simulink model "Neurofeedback_Draft_Models"  (R2022a)
settings: Solver=VariableStepAuto  StartTime=0.0  StopTime=10.0  RelTol=1e-3
settings Model: Creator=mariodelossantos  LastModifiedBy=mdls3

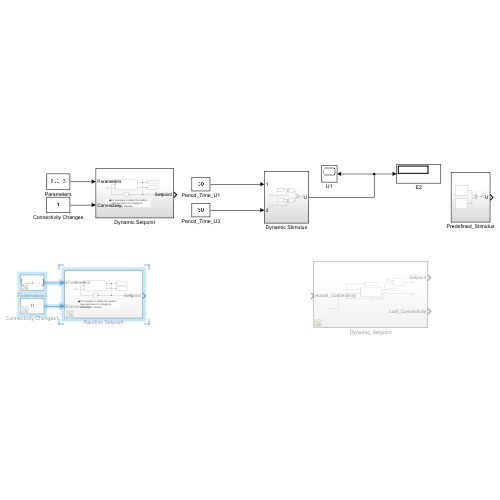
[thumbnail: Simulink's stored preview of the top-level diagram]
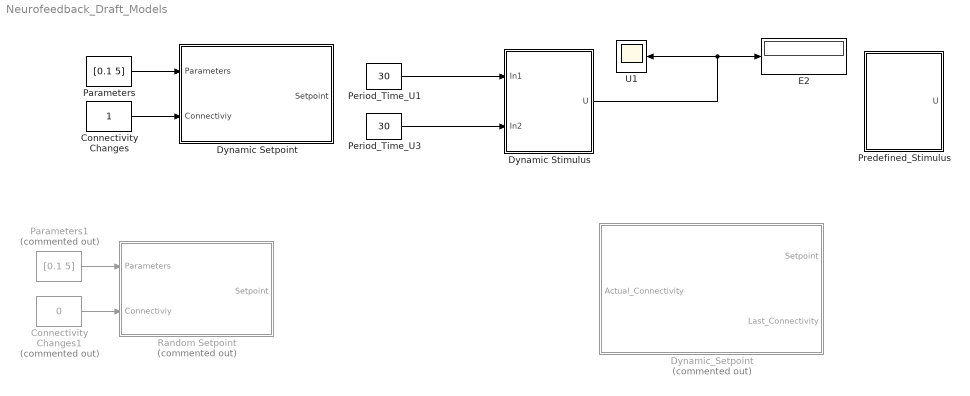
== system Neurofeedback_Draft_Models ==
  Connectivity Changes : Constant
  Connectivity Changes1 : Constant  Commented=on  Value=0
  Dynamic Setpoint : Subsystem
  Dynamic Stimulus : Subsystem
  Dynamic_Setpoint : Subsystem  Commented=on
  E2 : Display
  Parameters : Constant  Value=[0.1 5]
  Parameters1 : Constant  Commented=on  Value=[0.1 5]
  Period_Time_U1 : Constant  Value=30
  Period_Time_U3 : Constant  Value=30
  Predefined_Stimulus : Subsystem
  Random Setpoint : Subsystem  Commented=on
  U1 : Scope
  wires:
  Parameters/1 -> Dynamic Setpoint/1(Parameters)
  Connectivity Changes/1 -> Dynamic Setpoint/2(Connectiviy)
  Period_Time_U1/1 -> Dynamic Stimulus/1(In1)
  Period_Time_U3/1 -> Dynamic Stimulus/2(In2)
  Dynamic Stimulus/1(U) -> E2/1, U1/1
  Connectivity Changes1/1 -> Random Setpoint/2(Connectiviy)
  Parameters1/1 -> Random Setpoint/1(Parameters)

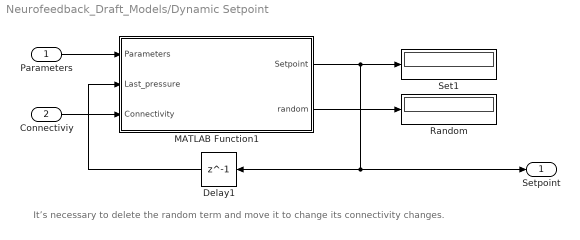
== system Neurofeedback_Draft_Models/Dynamic Setpoint ==
  note: It’s necessary to delete the random term and move it to change its connectivity changes.
  Parameters : Inport
  Connectiviy : Inport  Port=2
  Delay1 : Delay  DelayLength=1  InitialCondition=0
  MATLAB Function1 : MATLAB Function  TreatAsAtomicUnit=on
  Random : Display
  Set1 : Display
  Setpoint : Outport
  wires:
  Parameters/1 -> MATLAB Function1/1(Parameters)
  MATLAB Function1/2(random) -> Random/1
  MATLAB Function1/1(Setpoint) -> Set1/1, Setpoint/1, Delay1/1
  Delay1/1 -> MATLAB Function1/2(Last_pressure)
  Connectiviy/1 -> MATLAB Function1/3(Connectivity)

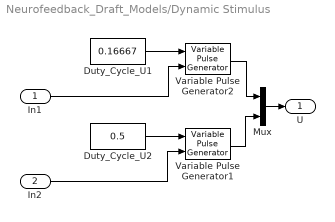
== system Neurofeedback_Draft_Models/Dynamic Stimulus ==
  In1 : Inport
  In2 : Inport  Port=2
  Duty_Cycle_U1 : Constant  Value=0.16667  OutMin=[0]  OutMax=[0.8]
  Duty_Cycle_U2 : Constant  Value=0.5  OutMin=[0]  OutMax=[0.8]
  Mux : Mux  Inputs=2
  Variable Pulse Generator1 : VariablePulseGenerator  RunAtFixedTimeIntervals=on  SampleTime=1/100
  Variable Pulse Generator2 : VariablePulseGenerator  RunAtFixedTimeIntervals=on  SampleTime=1/100
  U : Outport
  wires:
  In1/1 -> Variable Pulse Generator2/2
  Mux/1 -> U/1
  Variable Pulse Generator2/1 -> Mux/1
  Duty_Cycle_U1/1 -> Variable Pulse Generator2/1
  Duty_Cycle_U2/1 -> Variable Pulse Generator1/1
  In2/1 -> Variable Pulse Generator1/2
  Variable Pulse Generator1/1 -> Mux/2

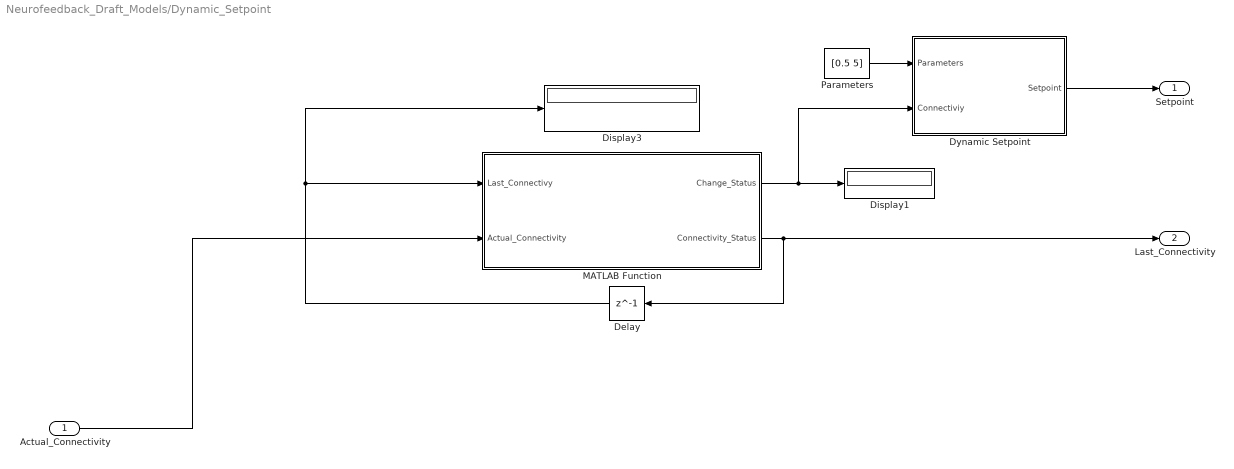
== system Neurofeedback_Draft_Models/Dynamic_Setpoint ==
  Actual_Connectivity : Inport
  Delay : Delay  DelayLength=1
  Display1 : Display
  Display3 : Display
  Dynamic Setpoint : Subsystem
  MATLAB Function : MATLAB Function  TreatAsAtomicUnit=on
  Parameters : Constant  Value=[0.5 5]
  Setpoint : Outport
  Last_Connectivity : Outport  Port=2
  wires:
  Dynamic Setpoint/1(Setpoint) -> Setpoint/1
  Actual_Connectivity/1 -> MATLAB Function/2(Actual_Connectivity)
  MATLAB Function/2(Connectivity_Status) -> Last_Connectivity/1, Delay/1
  Delay/1 -> Display3/1, MATLAB Function/1(Last_Connectivy)
  Parameters/1 -> Dynamic Setpoint/1(Parameters)
  MATLAB Function/1(Change_Status) -> Dynamic Setpoint/2(Connectiviy), Display1/1

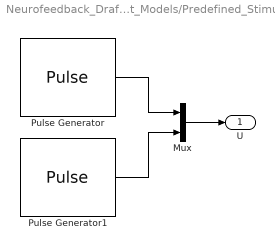
== system Neurofeedback_Draft_Models/Predefined_Stimulus ==
  Mux : Mux  Inputs=2
  Pulse Generator : DiscretePulseGenerator  Amplitude=0.6  Period=30  PulseWidth=5
  Pulse Generator1 : DiscretePulseGenerator  Amplitude=0.6  Period=30  PulseWidth=6
  U : Outport
  wires:
  Mux/1 -> U/1
  Pulse Generator/1 -> Mux/1
  Pulse Generator1/1 -> Mux/2

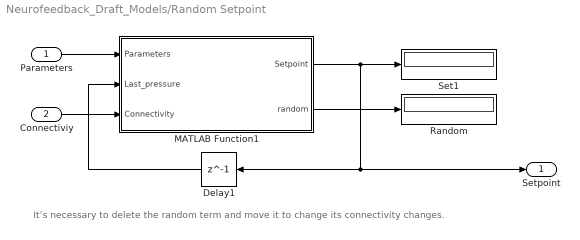
== system Neurofeedback_Draft_Models/Random Setpoint ==
  note: It’s necessary to delete the random term and move it to change its connectivity changes.
  Parameters : Inport
  Connectiviy : Inport  Port=2
  Delay1 : Delay  DelayLength=1  InitialCondition=0
  MATLAB Function1 : MATLAB Function  TreatAsAtomicUnit=on
  Random : Display
  Set1 : Display
  Setpoint : Outport
  wires:
  Parameters/1 -> MATLAB Function1/1(Parameters)
  MATLAB Function1/2(random) -> Random/1
  MATLAB Function1/1(Setpoint) -> Set1/1, Setpoint/1, Delay1/1
  Delay1/1 -> MATLAB Function1/2(Last_pressure)
  Connectiviy/1 -> MATLAB Function1/3(Connectivity)

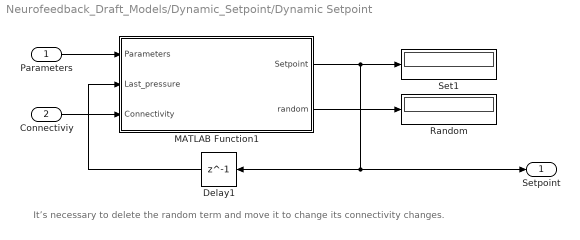
== system Neurofeedback_Draft_Models/Dynamic_Setpoint/Dynamic Setpoint ==
  note: It’s necessary to delete the random term and move it to change its connectivity changes.
  Parameters : Inport
  Connectiviy : Inport  Port=2
  Delay1 : Delay  DelayLength=1  InitialCondition=0
  MATLAB Function1 : MATLAB Function  TreatAsAtomicUnit=on
  Random : Display
  Set1 : Display
  Setpoint : Outport
  wires:
  Parameters/1 -> MATLAB Function1/1(Parameters)
  MATLAB Function1/2(random) -> Random/1
  MATLAB Function1/1(Setpoint) -> Set1/1, Setpoint/1, Delay1/1
  Delay1/1 -> MATLAB Function1/2(Last_pressure)
  Connectiviy/1 -> MATLAB Function1/3(Connectivity)

== matlab function Neurofeedback_Draft_Models/Random Setpoint/MATLAB Function1 ==
  settings: updateMethod=DISCRETE
  data: Setpoint output; Parameters input; Last_pressure input; random output; Connectivity input
function [Setpoint, random] = Random_Setpoint(Parameters, Last_pressure, Connectivity)
    %Parameters = [threshold Start_setpoint]
    temp = 0;
   %Pressure Setpoint selection
    pmin = 1;
    pmax = 10;
    new_pressure = pmin + rand(1)*(pmax-pmin);

    %Random used to simulate the connectivity changes, so we must change
    %the pressure setpoint when changes in the connectitvy are observed.
    min = 0;
    tmax = 10;
        %We should fine a random criteria to change the setpoint, not just
        %time, or the moment B changes. For now works to demostrate the
        %control without fNIRS
    random = min + rand(1) * (tmax - min) * new_pressure;
    if (Connectivity == 1)
         if (random < Parameters(1))
            %disp("Time")
            %disp(Time)
            temp = new_pressure;
            %disp("Setpoint")
            %disp(temp)
        else 
            temp = Last_pressure;
                if (Parameters(2) == temp || temp == 0)
                    temp = Parameters(2);
                else
                    temp = Last_pressure;
                end
         end  
    else
        temp = Parameters(2);
    end

    Setpoint = temp;

== matlab function Neurofeedback_Draft_Models/Dynamic_Setpoint/Dynamic Setpoint/MATLAB Function1 ==
  settings: updateMethod=DISCRETE
  data: Setpoint output; Parameters input; Last_pressure input; random output; Connectivity input
function [Setpoint, random] = Random_Setpoint(Parameters, Last_pressure, Connectivity)
    %Parameters = [threshold Start_setpoint]
    temp = 0;
   %Pressure Setpoint selection
    pmin = 5;
    pmax = 8;
    new_pressure = pmin + rand(1)*(pmax-pmin);

    %Random used to simulate the connectivity changes, so we must change
    %the pressure setpoint when changes in the connectitvy are observed.
    min = 0;
    tmax = 10;
        %We should fine a random criteria to change the setpoint, not just
        %time, or the moment B changes. For now works to demostrate the
        %control without fNIRS
    random = min + rand(1) * (tmax - min) * new_pressure;
    if (Connectivity == 1)
         if (random < Parameters(1))
            %disp("Time")
            %disp(Time)
            temp = new_pressure;
            %disp("Setpoint")
            %disp(temp)
        else 
            temp = Last_pressure;
                if (Parameters(2) == temp || temp == 0)
                    temp = Parameters(2);
                else
                    temp = Last_pressure;
                end
         end
    else
        temp = Last_pressure;
    end

    Setpoint = temp;

== matlab function Neurofeedback_Draft_Models/Dynamic Setpoint/MATLAB Function1 ==
  settings: updateMethod=DISCRETE
  data: Setpoint output; Parameters input; Last_pressure input; random output; Connectivity input
function [Setpoint, random] = Random_Setpoint(Parameters, Last_pressure, Connectivity)
    %Parameters = [threshold Start_setpoint]
    temp = 0;
   %Pressure Setpoint selection
    pmin = 5;
    pmax = 8;
    new_pressure = pmin + rand(1)*(pmax-pmin);

    %Random used to simulate the connectivity changes, so we must change
    %the pressure setpoint when changes in the connectitvy are observed.
    min = 0;
    tmax = 10;
        %We should fine a random criteria to change the setpoint, not just
        %time, or the moment B changes. For now works to demostrate the
        %control without fNIRS
    random = min + rand(1) * (tmax - min) * new_pressure;
    if (Connectivity == 1)
         if (random < Parameters(1))
            %disp("Time")
            %disp(Time)
            temp = new_pressure;
            %disp("Setpoint")
            %disp(temp)
        else 
            temp = Last_pressure;
                if (Parameters(2) == temp || temp == 0)
                    temp = Parameters(2);
                else
                    temp = Last_pressure;
                end
         end  
    else
        temp = Parameters(2);
    end

    Setpoint = temp;

== matlab function Neurofeedback_Draft_Models/Dynamic_Setpoint/MATLAB Function ==
  data: Last_Connectivy input boolean; Change_Status output; Actual_Connectivity input; Connectivity_Status output
function [Change_Status, Connectivity_Status] = Connectivity_Changes(Last_Connectivy , Actual_Connectivity)

if(Actual_Connectivity == Last_Connectivy)
    Change_Status = 0;
    
else
    Change_Status = 1;
end

Connectivity_Status = Actual_Connectivity;
